simulink subsystem "Battery"  (R2022b)
settings: Solver=VariableStepAuto  StartTime=0.0  StopTime=10.0  RelTol=1e-3
undefined symbols (not defined in the file): PlntBattCapInit, PlntBattChrgMax, PlntBattNumCellSer, PlntBattOpenCirctVolt, PlntBattVoltSocBpt
libraries: autolibdatasheetbattery x1
settings Model: ModifiedByFormat=The MathWorks, Inc.  Creator=The MathWorks, Inc.  LastModifiedBy=The MathWorks, Inc.
settings SolverCC: MaxZcPerStep=1
settings DebuggingCC: UnconnectedInputMsg=warning  UnconnectedOutputMsg=warning  UnconnectedLineMsg=warning
settings ModelReferenceCC: EnableRefExpFcnMdlSchedulingChecks=on
settings RTWCC: DLArmComputeVersion=19.05

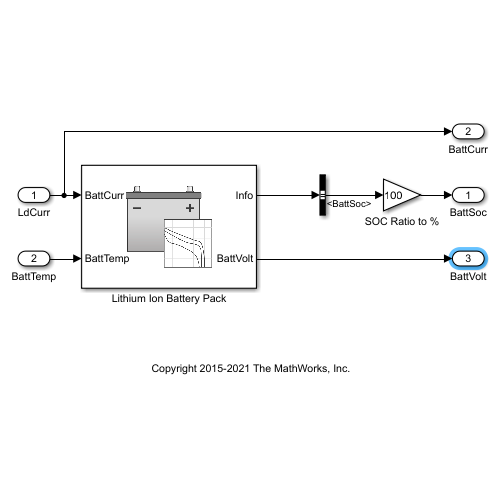
[thumbnail: Simulink's stored preview of the top-level diagram]
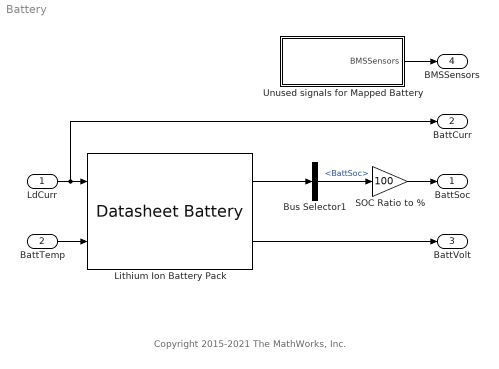
== system Battery ==
  note: Copyright 2015-2021 The MathWorks, Inc.
  LdCurr : Inport
  BattTemp : Inport  Port=2
  Bus Selector1 : BusSelector  OutputSignals=BattSoc
  Lithium Ion Battery Pack : autolibdatasheetbattery/Datasheet Battery  CapacityCtrl=Parameter  OutputVlt=Filtered  BattChargeMax=PlntBattChrgMax  Em=PlntBattOpenCirctVolt  CapLUTBp=PlntBattVoltSocBpt  RInt=PlntBattIntrnRes  BattTempBp=PlntBattTempBpt  CapSOCBp=PlntBattSocBpt  Ns=PlntBattNumCellSer  Np=PlntBattNumCellPar  BattCapInit=PlntBattCapInit  Tc=PlntBattTimeCnst  Vinit=PlntBattNumCellSer*interp1(PlntBattVoltSocBpt, PlntBattOpenCirctVolt, PlntBattCapInit/PlntBattChrgMax)  RefBlkName='autolibdatasheetbattery/Datasheet Battery'
  SOC Ratio to % : Gain  Gain=100
  Unused signals for Mapped Battery : Subsystem
  BattSoc : Outport  VectorParamsAs1DForOutWhenUnconnected=off
  BattCurr : Outport  Port=2  VectorParamsAs1DForOutWhenUnconnected=off
  BattVolt : Outport  Port=3  VectorParamsAs1DForOutWhenUnconnected=off
  BMSSensors : Outport  Port=4  VectorParamsAs1DForOutWhenUnconnected=off
  wires:
  Lithium Ion Battery Pack/2 -> BattVolt/1
  BattTemp/1 -> Lithium Ion Battery Pack/2
  Bus Selector1/1 -> SOC Ratio to %/1  "<BattSoc>"
  LdCurr/1 -> BattCurr/1, Lithium Ion Battery Pack/1
  SOC Ratio to %/1 -> BattSoc/1
  Lithium Ion Battery Pack/1 -> Bus Selector1/1
  Unused signals for Mapped Battery/1(BMSSensors) -> BMSSensors/1

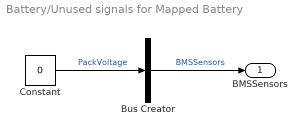
== system Battery/Unused signals for Mapped Battery ==
  Bus Creator : BusCreator  Inputs=1
  Constant : Constant  Value=0  SampleTime=-1
  BMSSensors : Outport
  wires:
  Constant/1 -> Bus Creator/1  "PackVoltage"
  Bus Creator/1 -> BMSSensors/1  "BMSSensors"
